simulink model "schemat_dyskretny"  (R2022a)
settings: Solver=VariableStepAuto  StartTime=0.0  StopTime=100  RelTol=1e-3
values from neighbouring files (symbols this model uses):
  K = 3    [dane.m]    (also in k_stat.m = (111*ul)/50 - (171*ul.^2)/100 - (12*ul.^3)/5 + 117/100; untitled.m)
  L1 = 0.39    [dane.m]    (also in untitled.m)
  L2 = 0.37    [dane.m]    (also in untitled.m)
  L3 = -0.19    [dane.m]    (also in untitled.m)
  L4 = -0.2    [dane.m]    (also in untitled.m)
  T1 = 6    [dane.m]    (also in untitled.m)
  T2 = 7    [dane.m]    (also in untitled.m)
  Tp = 1    [dane.m]    (also in untitled.m)
  ul = -0.1    [dane.m]    (also in k_stat.m = -1:0.1:1; wykresy.m = -0.5)
settings Model: Creator=danie  LastModifiedBy=danie

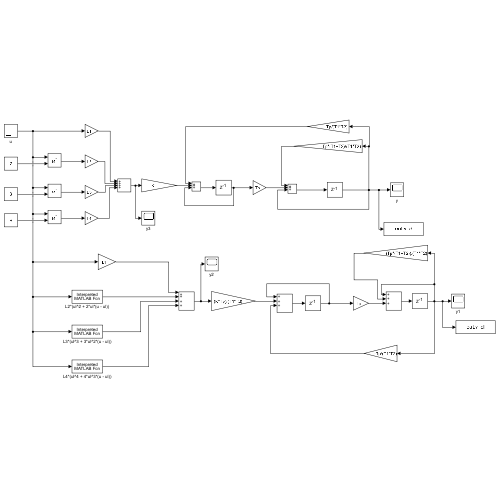
[thumbnail: Simulink's stored preview of the top-level diagram]
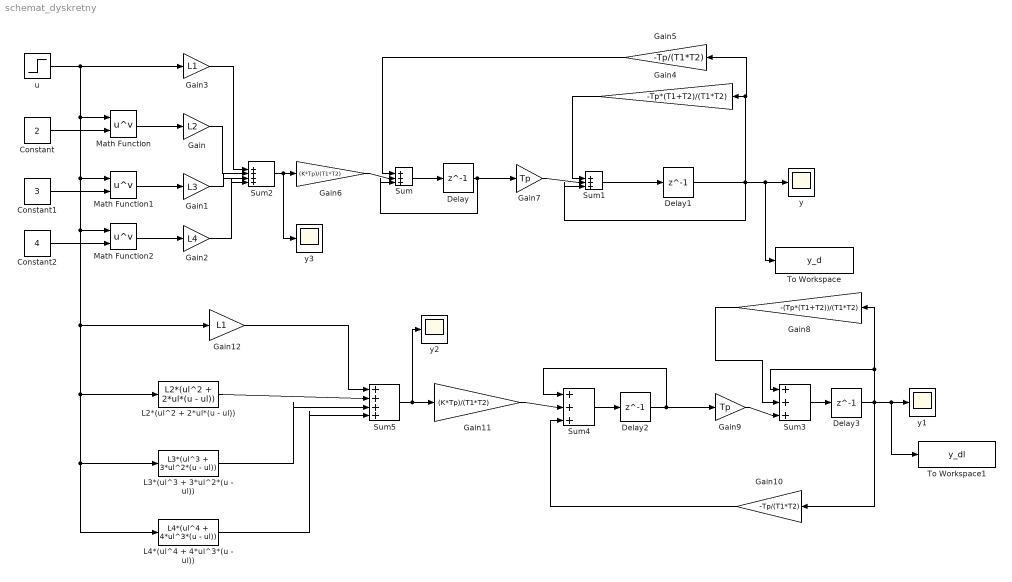
== system schemat_dyskretny ==
  Constant : Constant  Value=2
  Constant1 : Constant  Value=3
  Constant2 : Constant  Value=4
  Delay{,1..3} (4 alike) : Delay  DelayLength=1  InitialCondition=0  SampleTime=Tp
  Gain : Gain  Gain=L2
  Gain1 : Gain  Gain=L3
  Gain10 : Gain  Gain=-Tp/(T1*T2)
  Gain11 : Gain  Gain=(K*Tp)/(T1*T2)
  Gain12 : Gain  Gain=L1
  Gain2 : Gain  Gain=L4
  Gain3 : Gain  Gain=L1
  Gain4 : Gain  Gain=-Tp*(T1+T2)/(T1*T2)
  Gain5 : Gain  Gain=-Tp/(T1*T2)
  Gain6 : Gain  Gain=(K*Tp)/(T1*T2)
  Gain7 : Gain  Gain=Tp
  Gain8 : Gain  Gain=-(Tp*(T1+T2))/(T1*T2)
  Gain9 : Gain  Gain=Tp
  L2*(ul^2 + 2*ul*(u - ul)) : MATLABFcn  MATLABFcn=L2*(ul^2 + 2*ul*(u - ul))
  L3*(ul^3 + 3*ul^2*(u - ul)) : MATLABFcn  MATLABFcn=L3*(ul^3 + 3*ul^2*(u - ul))
  L4*(ul^4 + 4*ul^3*(u - ul)) : MATLABFcn  MATLABFcn=L4*(ul^4 + 4*ul^3*(u - ul))
  Math Function : Math  Operator=pow
  Math Function1 : Math  Operator=pow
  Math Function2 : Math  Operator=pow
  Sum{,1,3..4} (4 alike) : Sum  Inputs=+++|
  Sum2 : Sum  Inputs=++++|
  Sum5 : Sum  Inputs=++++|
  To Workspace : ToWorkspace  VariableName=y_d  SaveFormat=Structure With Time  SampleTime=Tp
  To Workspace1 : ToWorkspace  VariableName=y_dl  SaveFormat=Structure With Time  SampleTime=Tp
  u : Step  SampleTime=0
  y{,1..3} (4 alike) : Scope
  wires:
  Gain/1 -> Sum2/2
  Gain2/1 -> Sum2/4
  Gain3/1 -> Sum2/1
  Delay1/1 -> Sum1/3, Gain4/1, Gain5/1, To Workspace/1, y/1
  Constant2/1 -> Math Function2/2
  Constant/1 -> Math Function/2
  Math Function1/1 -> Gain1/1
  Sum2/1 -> y3/1, Gain6/1
  Math Function/1 -> Gain/1
  Gain6/1 -> Sum/2
  Constant1/1 -> Math Function1/2
  Gain5/1 -> Sum/1
  Gain4/1 -> Sum1/1
  Math Function2/1 -> Gain2/1
  Gain1/1 -> Sum2/3
  Sum1/1 -> Delay1/1
  Sum/1 -> Delay/1
  Delay/1 -> Sum/3, Gain7/1
  Gain7/1 -> Sum1/2
  L3*(ul^3 + 3*ul^2*(u - ul))/1 -> Sum5/3
  Gain12/1 -> Sum5/1
  Sum5/1 -> y2/1, Gain11/1
  Gain11/1 -> Sum4/2
  Delay3/1 -> Gain10/1, To Workspace1/1, y1/1, Gain8/1, Sum3/1
  Gain8/1 -> Sum3/2
  Delay2/1 -> Sum4/1, Gain9/1
  L4*(ul^4 + 4*ul^3*(u - ul))/1 -> Sum5/4
  Sum4/1 -> Delay2/1
  Gain9/1 -> Sum3/3
  Gain10/1 -> Sum4/3
  L2*(ul^2 + 2*ul*(u - ul))/1 -> Sum5/2
  Sum3/1 -> Delay3/1
  u/1 -> Gain3/1, L2*(ul^2 + 2*ul*(u - ul))/1, L3*(ul^3 + 3*ul^2*(u - ul))/1, L4*(ul^4 + 4*ul^3*(u - ul))/1, Gain12/1, Math Function2/1, Math Function1/1, Math Function/1
